simulink model "testburner"  (R2012b)
settings: Solver=ode45  StartTime=0.0  StopTime=10.0  RelTol=1e-3
settings Model: Creator=tlavelle  LastModifiedBy=tlavelle

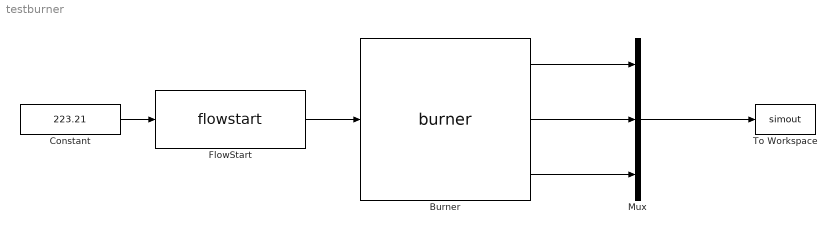
== system testburner ==
  "Burner " : M-S-Function  FunctionName=burner  Parameters=Wfuel,hFuel,dP  mask{Wfuel=.02224, hFuel=-700, dP=.055}
      mask prompts: Wfuel "FAR"; hFuel "Fuel enthalpy"
      mask Display:
      | color('red'); port_label('input',1,'Flow In')
      | color('red'); port_label('output',1,'Flow Out')
      | 
      | color('green'); port_label('output',2,'Wfuel')
  Constant : Constant  Value=223.21
  FlowStart : M-S-Function  FunctionName=flowstart  Parameters=Tt,Pt,comp1,comp2,comp3,comp4,comp5,comp6  mask{Tt=1398, Pt=297.127, comp1=1, comp2=0, comp3=0, comp4=0, comp5=0, comp6=0}
      mask prompts: Tt "Exit Temperature"; Pt "Exit Pressure"
      mask Display:
      | color('red'); port_label('input',1,'Flow')
      | color('red'); port_label('output',1,'Flow Out')
  Mux : Mux  Inputs=3
  To Workspace : ToWorkspace  VariableName=simout  SampleTime=-1  SaveFormat=Timeseries
  wires:
  Constant/1 -> FlowStart/1
  FlowStart/1 -> "Burner "/1
  "Burner "/1 -> Mux/1
  "Burner "/2 -> Mux/2
  Mux/1 -> To Workspace/1
  "Burner "/3 -> Mux/3
